simulink model "simulink_model"  (R2019a)
settings: Solver=ode3  StartTime=0.0  StopTime=15  FixedStep=1e-4  RelTol=1e-3  EnableMultiTasking=on
values from neighbouring files (symbols this model uses):
  Bv = 0.003    [bldc_params.m]
  J = 0.012    [bldc_params.m]
  Ke_2phase = 0.11    [bldc_params.m]
  Kt_2phase = 0.11    [bldc_params.m]
  L_2phase = 0.30    (= 0.3)    [bldc_params.m]
  R_2phase = 0.16    [bldc_params.m]
  V = [L_2phase.*J, (R_2phase*J+L_2phase.*Bv),(R_2phase*Bv+Kt_2phase.*Ke_2phase)]    [bldc_params.m]
  W = Kt_2phase    (= 0.11)    [bldc_params.m]
libraries: simulink x2
settings Model: Creator=ayyrao  LastModifiedBy=Nelson Manuel
settings DataIOCC: LimitDataPoints=on  SaveFormat=Array  ReturnWorkspaceOutputs=off
settings OptimizationCC: LifeSpan=inf
settings DebuggingCC: SFUnexpectedBacktrackingDiag=warning  SFNoUnconditionalDefaultTransitionDiag=warning  SFExecutionAtInitializationDiag=none  ArithmeticOperatorsInVariantConditions=warning
settings HardwareCC: ProdBitPerPointer=32  ProdBitPerSizeT=32  ProdBitPerPtrDiffT=32  ProdLargestAtomicFloat=None  ProdIntDivRoundTo=Undefined  ProdEndianess=Unspecified  ProdWordSize=32  ProdHWDeviceType=32-bit Generic
settings ModelReferenceCC: PropagateSignalLabelsOutOfModel=off
settings SFSimCC: SimUseLocalCustomCode=off
settings RTWCC: RTWUseLocalCustomCode=off
settings CodeAppCC: StateflowObjectComments=on
settings GRTTargetCC: TargetLangStandard=C89/C90 (ANSI)  GeneratePreprocessorConditionals=Disable all
settings ConfigComp: CovMetricSettings=dw  CovHtmlReporting=on  CovSaveCumulativeToWorkspaceVar=on  CovSaveSingleToWorkspaceVar=on  CovExternalEMLEnable=off

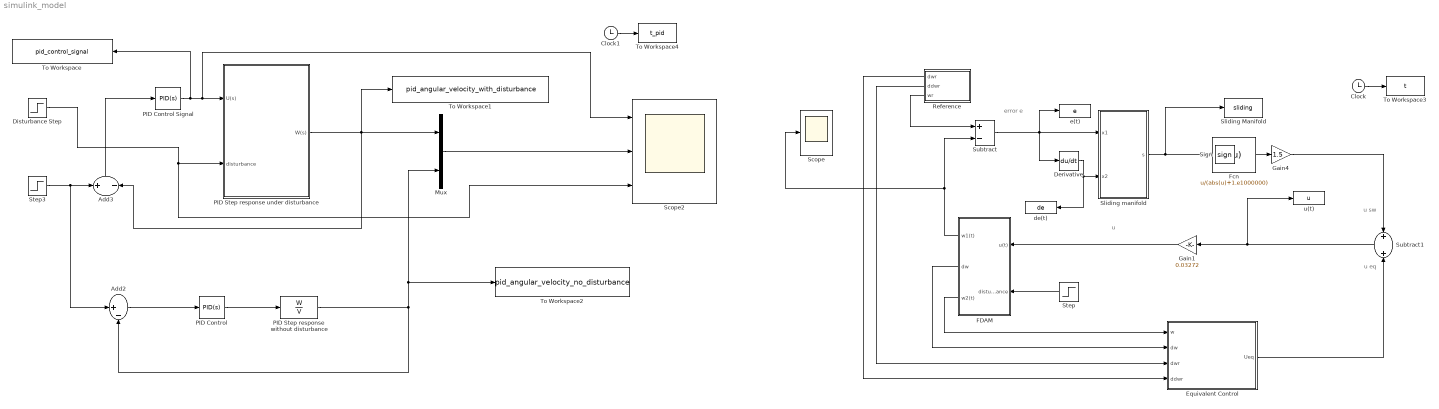
== system simulink_model ==
  note: error e
  note: u
  note: u sw
  note: u eq
  Add2 : Sum  Inputs=|+-
  Add3 : Sum  Inputs=+-
  Clock : Clock
  Clock1 : Clock
  Derivative : Derivative
  Disturbance Step : Step  Time=5  After=0.1  SampleTime=0
  Equivalent Control : MATLAB Function  TreatAsAtomicUnit=on
  FDAM : Subsystem
  Fcn : Fcn  Expr=u/(abs(u)+1.e1000000)
      mask Display: image('D:\KKU\KİŞİSEL KÜTÜPHANE\Elektrik Motorlarının Denetim\Makale\Kitap\Sliding Mode Control\Odaklamak\sigmoid.PNG');
  Gain1 : Gain  Gain=0.03272
  Gain4 : Gain  Gain=1.5
  Mux : Mux  Inputs=2
  PID Control : simulink/Continuous/PID Controller  Controller=PID  Form=Parallel  TimeDomain=Continuous-time  SampleTime=-1  IntegratorMethod=Forward Euler  FilterMethod=Forward Euler  ControllerParametersSource=internal  P=4.43118956360769  I=5.42773395929543  D=0.898374810186208  UseFilter=on  N=3179.70625454392  TunerSelectOption=Transfer Function Based (PID Tuner App)  InitialConditionSource=internal  InitialConditionForIntegrator=0  InitialConditionForFilter=0  DifferentiatorICPrevScaledInput=0  ExternalReset=none  TrackingMode=off  Kt=1  LimitOutput=off  UpperSaturationLimit=inf  LowerSaturationLimit=-inf  LinearizeAsGain=on  AntiWindupMode=none  Kb=1  POutMin=[]  POutMax=[]  IOutMin=[]  IOutMax=[]  DOutMin=[]  DOutMax=[]  NOutMin=[]  NOutMax=[]  SumOutMin=[]  SumOutMax=[]  SaturationOutMin=[]  SaturationOutMax=[]  PParamMin=[]  PParamMax=[]  IParamMin=[]  IParamMax=[]  DParamMin=[]  DParamMax=[]  NParamMin=[]  NParamMax=[]  KbParamMin=[]  KbParamMax=[]  KtParamMin=[]  KtParamMax=[]  KbOutMin=[]  KbOutMax=[]  KtOutMin=[]  KtOutMax=[]  IntegratorOutMin=[]  IntegratorOutMax=[]  FilterOutMin=[]  FilterOutMax=[]  SumI1OutMin=[]  SumI1OutMax=[]  SumI2OutMin=[]  SumI2OutMax=[]  SumI3OutMin=[]  SumI3OutMax=[]  SumI4OutMin=[]  SumI4OutMax=[]  SumDOutMin=[]  SumDOutMax=[]  DifferentiatorOutMin=[]  DifferentiatorOutMax=[]  FilterDiffOutCoefMin=[]  FilterDiffOutCoefMax=[]  ReciprocalOutMin=[]  ReciprocalOutMax=[]  SumDenOutMin=[]  SumDenOutMax=[]  SumNumOutMin=[]  SumNumOutMax=[]  DivideOutMin=[]  DivideOutMax=[]  IntegratorContinuousStateAttributes=''  IntegratorStateMustResolveToSignalObject=off  IntegratorRTWStateStorageClass=Auto  FilterContinuousStateAttributes=''  FilterStateMustResolveToSignalObject=off  FilterRTWStateStorageClass=Auto  ParallelPVariant=InternalParameters  IdealPVariant=Disabled  IVariant=InternalParameters  DVariant=InternalParameters  IntegratorVariant=Continuous  SatVariant=Disabled  AWVariant=Passthrough  PCopyVariant=Disabled  TRVariant=Disabled  FdbkBlocksVariant=Forward  IdealPFdbkVariant=Disabled  SatFdbkVariant=Disabled  DerivativeFilterVariant=ContFilter  NVariant=InternalParameters  NCopyVariant=Disabled  FilterICVariant=InternalICsFilter  IntegratorICVariant=InternalICs  ExternalResetVariant=Disabled  TRSumVariant=Passthrough  SumFdbkVariant=Disabled  SumVariant=Sum_PID
  PID Control Signal : simulink/Continuous/PID Controller  Controller=PID  Form=Parallel  TimeDomain=Continuous-time  SampleTime=-1  IntegratorMethod=Forward Euler  FilterMethod=Forward Euler  ControllerParametersSource=internal  P=4.43118956360769  I=5.42773395929543  D=0.898374810186208  UseFilter=on  N=3179.70625454392  TunerSelectOption=Transfer Function Based (PID Tuner App)  InitialConditionSource=internal  InitialConditionForIntegrator=0  InitialConditionForFilter=0  DifferentiatorICPrevScaledInput=0  ExternalReset=none  TrackingMode=off  Kt=1  LimitOutput=off  UpperSaturationLimit=inf  LowerSaturationLimit=-inf  LinearizeAsGain=on  AntiWindupMode=none  Kb=1  POutMin=[]  POutMax=[]  IOutMin=[]  IOutMax=[]  DOutMin=[]  DOutMax=[]  NOutMin=[]  NOutMax=[]  SumOutMin=[]  SumOutMax=[]  SaturationOutMin=[]  SaturationOutMax=[]  PParamMin=[]  PParamMax=[]  IParamMin=[]  IParamMax=[]  DParamMin=[]  DParamMax=[]  NParamMin=[]  NParamMax=[]  KbParamMin=[]  KbParamMax=[]  KtParamMin=[]  KtParamMax=[]  KbOutMin=[]  KbOutMax=[]  KtOutMin=[]  KtOutMax=[]  IntegratorOutMin=[]  IntegratorOutMax=[]  FilterOutMin=[]  FilterOutMax=[]  SumI1OutMin=[]  SumI1OutMax=[]  SumI2OutMin=[]  SumI2OutMax=[]  SumI3OutMin=[]  SumI3OutMax=[]  SumI4OutMin=[]  SumI4OutMax=[]  SumDOutMin=[]  SumDOutMax=[]  DifferentiatorOutMin=[]  DifferentiatorOutMax=[]  FilterDiffOutCoefMin=[]  FilterDiffOutCoefMax=[]  ReciprocalOutMin=[]  ReciprocalOutMax=[]  SumDenOutMin=[]  SumDenOutMax=[]  SumNumOutMin=[]  SumNumOutMax=[]  DivideOutMin=[]  DivideOutMax=[]  IntegratorContinuousStateAttributes=''  IntegratorStateMustResolveToSignalObject=off  IntegratorRTWStateStorageClass=Auto  FilterContinuousStateAttributes=''  FilterStateMustResolveToSignalObject=off  FilterRTWStateStorageClass=Auto  ParallelPVariant=InternalParameters  IdealPVariant=Disabled  IVariant=InternalParameters  DVariant=InternalParameters  IntegratorVariant=Continuous  SatVariant=Disabled  AWVariant=Passthrough  PCopyVariant=Disabled  TRVariant=Disabled  FdbkBlocksVariant=Forward  IdealPFdbkVariant=Disabled  SatFdbkVariant=Disabled  DerivativeFilterVariant=ContFilter  NVariant=InternalParameters  NCopyVariant=Disabled  FilterICVariant=InternalICsFilter  IntegratorICVariant=InternalICs  ExternalResetVariant=Disabled  TRSumVariant=Passthrough  SumFdbkVariant=Disabled  SumVariant=Sum_PID
  PID Step response under disturbance : Subsystem
  PID Step response without disturbance : TransferFcn  Numerator=W  Denominator=V
  Reference : Subsystem
  Scope : Scope
  Scope2 : Scope  NumInputPorts=3
  Sign : Signum
  Sliding Manifold : ToWorkspace  VariableName=sliding  SampleTime=-1
  Sliding manifold : MATLAB Function  TreatAsAtomicUnit=on
  Step : Step  Time=5  After=0.01  SampleTime=0
  Step3 : Step  Time=0  SampleTime=0
  Subtract : Sum  Inputs=+-
  Subtract1 : Sum
  To Workspace : ToWorkspace  VariableName=pid_control_signal  SampleTime=-1
  To Workspace1 : ToWorkspace  VariableName=pid_angular_velocity_with_disturbance  SampleTime=-1
  To Workspace2 : ToWorkspace  VariableName=pid_angular_velocity_no_disturbance  SampleTime=-1
  To Workspace3 : ToWorkspace  VariableName=t  SampleTime=-1
  To Workspace4 : ToWorkspace  VariableName=t_pid  SampleTime=-1
  de(t) : ToWorkspace  VariableName=de  SampleTime=-1
  e(t) : ToWorkspace  VariableName=e  SampleTime=-1
  u(t) : ToWorkspace  VariableName=u  SampleTime=-1
  wires:
  Clock/1 -> To Workspace3/1
  Sign/1 -> Gain4/1
  Sliding manifold/1(s) -> Sign/1, Sliding Manifold/1
  Reference/3(wr) -> Subtract/1
  Subtract/1 -> e(t)/1, Sliding manifold/1(x1), Derivative/1
  Gain4/1 -> Subtract1/1
  Subtract1/1 -> u(t)/1, Gain1/1
  Gain1/1 -> FDAM/1(u(t))
  Equivalent Control/1(Ueq) -> Subtract1/2
  FDAM/2(dw) -> Equivalent Control/2(dw)
  FDAM/1(w1(t)) -> Scope/1, Subtract/2
  FDAM/3(w2(t)) -> Equivalent Control/1(w)
  Reference/2(ddwr) -> Equivalent Control/3(dwr)
  Reference/1(dwr) -> Equivalent Control/4(ddwr)
  Derivative/1 -> de(t)/1, Sliding manifold/2(x2)
  Step/1 -> FDAM/2(disturbance)
  PID Step response without disturbance/1 -> Mux/2, To Workspace2/1, Add2/2
  Clock1/1 -> To Workspace4/1
  PID Control Signal/1 -> To Workspace/1, Scope2/1, PID Step response under disturbance/1(U(s))
  PID Control/1 -> PID Step response without disturbance/1
  Disturbance Step/1 -> Scope2/3, PID Step response under disturbance/2(disturbance)
  Add2/1 -> PID Control/1
  Add3/1 -> PID Control Signal/1
  PID Step response under disturbance/1(W(s)) -> To Workspace1/1, Mux/1, Add3/2
  Step3/1 -> Add2/1, Add3/1
  Mux/1 -> Scope2/2

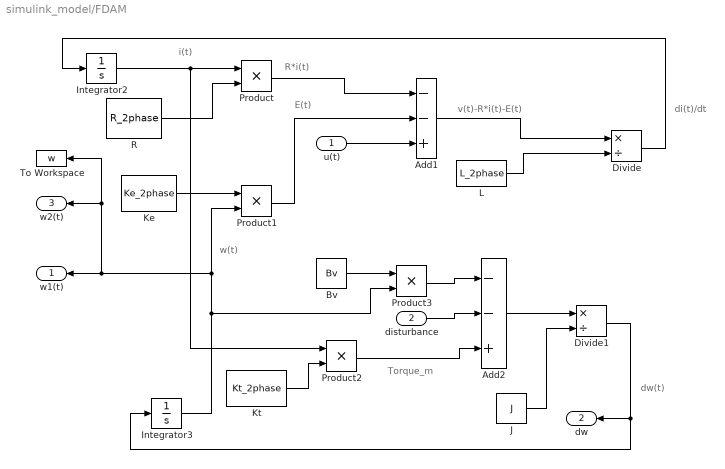
== system simulink_model/FDAM ==
  note: dw(t)
  note: i(t)
  note: di(t)/dt
  note: w(t)
  note: v(t)-R*i(t)-E(t)
  note: Torque_m
  note: E(t)
  note: R*i(t)
  u(t) : Inport
  disturbance : Inport  Port=2
  Add1 : Sum  Inputs=--+
  Add2 : Sum  Inputs=--+
  Bv : Constant  Value=Bv
  Divide : Product  Inputs=*/
  Divide1 : Product  Inputs=*/
  Integrator2 : Integrator
  Integrator3 : Integrator
  J : Constant  Value=J
  Ke : Constant  Value=Ke_2phase
  Kt : Constant  Value=Kt_2phase
  L : Constant  Value=L_2phase
  Product{,1..3} (4 alike) : Product
  R : Constant  Value=R_2phase
  To Workspace : ToWorkspace  VariableName=w  SampleTime=-1
  w1(t) : Outport
  dw : Outport  Port=2
  w2(t) : Outport  Port=3
  wires:
  Product1/1 -> Add1/2
  Bv/1 -> Product3/1
  L/1 -> Divide/2
  Product2/1 -> Add2/3
  Integrator2/1 -> Product2/1, Product/1
  Ke/1 -> Product1/1
  R/1 -> Product/2
  Kt/1 -> Product2/2
  Product3/1 -> Add2/1
  u(t)/1 -> Add1/3
  Product/1 -> Add1/1
  Add1/1 -> Divide/1
  J/1 -> Divide1/2
  Integrator3/1 -> Product1/2, w1(t)/1, To Workspace/1, w2(t)/1, Product3/2
  Divide/1 -> Integrator2/1
  Add2/1 -> Divide1/1
  Divide1/1 -> dw/1, Integrator3/1
  disturbance/1 -> Add2/2

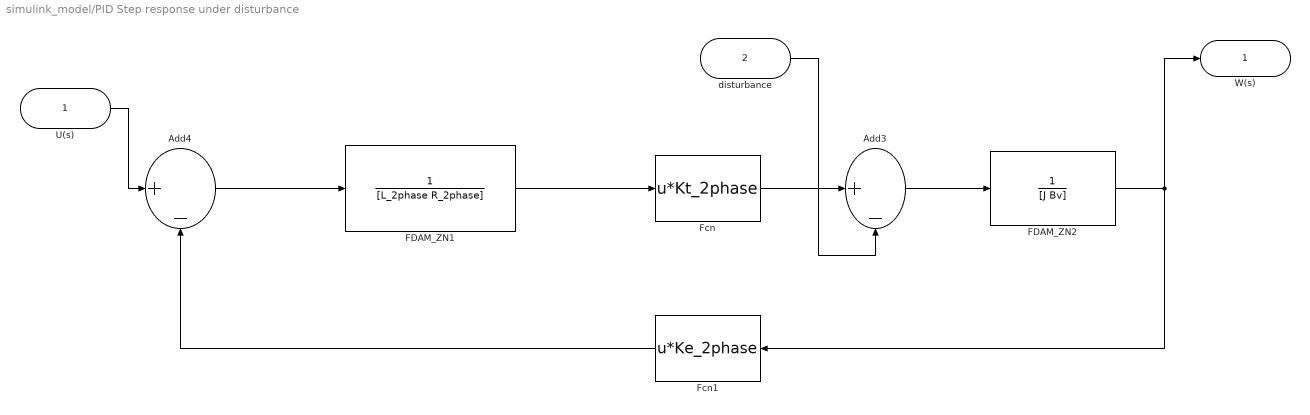
== system simulink_model/PID Step response under disturbance ==
  U(s) : Inport
  disturbance : Inport  Port=2
  Add3 : Sum  Inputs=|+-
  Add4 : Sum  Inputs=|+-
  FDAM_ZN1 : TransferFcn  Numerator=1  Denominator=[L_2phase R_2phase]
  FDAM_ZN2 : TransferFcn  Numerator=1  Denominator=[J Bv]
  Fcn : Fcn  Expr=u*Kt_2phase
  Fcn1 : Fcn  Expr=u*Ke_2phase
  W(s) : Outport
  wires:
  Fcn1/1 -> Add4/2
  Fcn/1 -> Add3/1
  Add3/1 -> FDAM_ZN2/1
  U(s)/1 -> Add4/1
  FDAM_ZN1/1 -> Fcn/1
  Add4/1 -> FDAM_ZN1/1
  FDAM_ZN2/1 -> W(s)/1, Fcn1/1
  disturbance/1 -> Add3/2

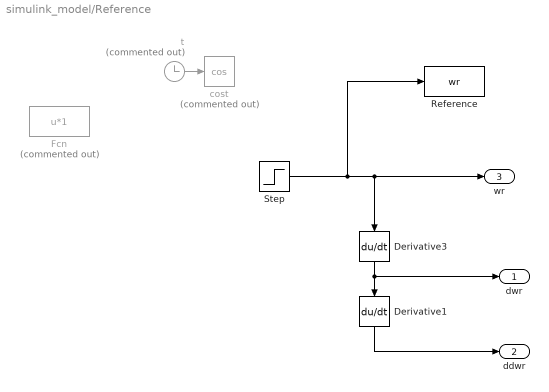
== system simulink_model/Reference ==
  Derivative1 : Derivative
  Derivative3 : Derivative
  Fcn : Fcn  Commented=on  Expr=u*1
  Reference : ToWorkspace  VariableName=wr  SampleTime=-1
  Step : Step  Time=0  SampleTime=0
  cost : Trigonometry  Commented=on  Operator=cos
  t : Clock  Commented=on
  dwr : Outport
  ddwr : Outport  Port=2
  wr : Outport  Port=3
  wires:
  Step/1 -> Reference/1, wr/1, Derivative3/1
  Derivative3/1 -> dwr/1, Derivative1/1
  Derivative1/1 -> ddwr/1
  t/1 -> cost/1

== matlab function simulink_model/Equivalent Control ==
  data: w input; dw input; Ueq output; dwr input; ddwr input
function Ueq = fcn(w,dw,dwr,ddwr)

lambda=1.5; % here lambda is 1.5
%Ueq=(M2+M3-lambda)*dw+(M2*M3+M4)*w+ddwr+lambda*dwr
Ueq =(0.78-lambda)*dw+3.49*w+ddwr+lambda*dwr; 
end

== matlab function simulink_model/Sliding manifold ==
  data: x1 input; s output; x2 input
function s = fcn(x1,x2)
%% Sliding manifold calculation
s =x2+1.5*x1; % here lambda is 1.5
end
